simulink model "sim_wocon"  (R2018a)
settings: Solver=FixedStepAuto  StartTime=0.0  StopTime=10.0  RelTol=1e-3
values from neighbouring files (symbols this model uses):
  a11 = -2*(cf+cr)/m/v    (= -9.36)    [dyc.m]    (also in dyc_obs.m; normal_vehicle.m)
  a12 = -1-2*(lf*cf-lr*cr)/m/v/v    (= -0.9745984)    [dyc.m]    (also in dyc_obs.m; normal_vehicle.m)
  a21 = -2*(lf*cf-lr*cr)/iz    (= 12.3270440252)    [dyc.m]    (also in dyc_obs.m; normal_vehicle.m)
  a22 = -2*(lf*lf*cf+lr*lr*cr)/iz/v    (= -9.16473962264)    [dyc.m]    (also in dyc_obs.m; normal_vehicle.m)
  b11 = 2*cf/m/v    (= 3.6)    [dyc.m]    (also in dyc_obs.m; normal_vehicle.m)
  b21 = 2*lf*cf/iz    (= 94.3396226415)    [dyc.m]    (also in dyc_obs.m; normal_vehicle.m)
  mydt = 0.01    [dyc.m]    (also in dyc_obs.m; normal_vehicle.m)
  n = 18.7    [dyc.m]    (also in dyc_obs.m; normal_vehicle.m)
settings Model: Creator=aoki-soya  LastModifiedBy=aoki-soya

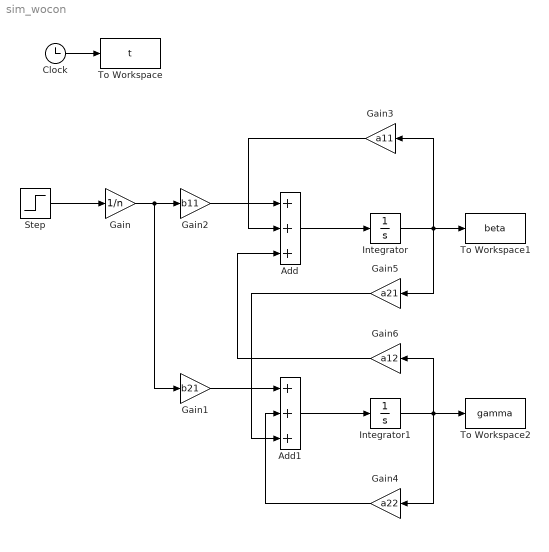
== system sim_wocon ==
  Add : Sum  Inputs=+++
  Add1 : Sum  Inputs=+++
  Clock : Clock
      settings: Decimation=1/mydt
  Gain : Gain  Gain=1/n
  Gain1 : Gain  Gain=b21
  Gain2 : Gain  Gain=b11
  Gain3 : Gain  Gain=a11
  Gain4 : Gain  Gain=a22
  Gain5 : Gain  Gain=a21
  Gain6 : Gain  Gain=a12
  Integrator : Integrator
  Integrator1 : Integrator
  Step : Step  After=15*pi/180  SampleTime=mydt
  To Workspace : ToWorkspace  VariableName=t  SaveFormat=Timeseries  SampleTime=-1
  To Workspace1 : ToWorkspace  VariableName=beta  SaveFormat=Timeseries  SampleTime=-1
  To Workspace2 : ToWorkspace  VariableName=gamma  SaveFormat=Timeseries  SampleTime=-1
  wires:
  Clock/1 -> To Workspace/1
  Step/1 -> Gain/1
  Gain/1 -> Gain1/1, Gain2/1
  Gain2/1 -> Add/1
  Add/1 -> Integrator/1
  Integrator/1 -> Gain5/1, Gain3/1, To Workspace1/1
  Gain3/1 -> Add/2
  Add1/1 -> Integrator1/1
  Integrator1/1 -> Gain6/1, Gain4/1, To Workspace2/1
  Gain4/1 -> Add1/2
  Gain1/1 -> Add1/1
  Gain5/1 -> Add1/3
  Gain6/1 -> Add/3
